simulink subsystem "egram_transmitter"  (R2020a)
settings: Solver=VariableStepAuto  StartTime=0.0  StopTime=10.0  RelTol=1e-3
libraries: etargetslib x2, frdmk64flib x1
settings Model: Creator=Ethan  LastModifiedBy=Ethan

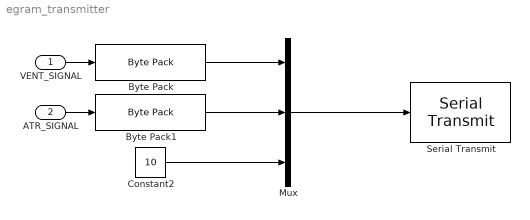
== system egram_transmitter ==
  VENT_SIGNAL : Inport
  ATR_SIGNAL : Inport  Port=2
  Byte Pack : etargetslib/Byte Pack  datatypes={'double'}  byteAlign=1
  Byte Pack1 : etargetslib/Byte Pack  datatypes={'double'}  byteAlign=1
  Constant2 : Constant  Value=10  OutDataTypeStr=uint8
  Mux : Mux  Inputs=3
  Serial Transmit : frdmk64flib/Serial Transmit  SCIModule=0  Baudrate=uint32(9600)  Parity=None  StopBits=1  HardwareFlowControl=None  ByteOrder=LittleEndian  BlockingMode=on  OutputStatus=off
  wires:
  ATR_SIGNAL/1 -> Byte Pack1/1
  VENT_SIGNAL/1 -> Byte Pack/1
  Byte Pack/1 -> Mux/1
  Constant2/1 -> Mux/3
  Byte Pack1/1 -> Mux/2
  Mux/1 -> Serial Transmit/1
